simulink model "spec_avg_CRD"  (R2025b)
settings: Solver=FixedStepDiscrete  StartTime=0.0  StopTime=0.0005  FixedStep=1/Fs  RelTol=1e-3
undefined symbols (not defined in the file): Add, chirp_counts, chirp_outputs, FFT_LENGTH, Fs, h, N, Shift, specAvg, T, Ts
libraries: hdlsllib x5, dsphdlsigops2 x3, dsphdlmathfun2 x1, commutil2 x1, dsphdlxfrm2 x1
settings Model: MinMaxOverflowLogging=MinMaxAndOverflow  FPTRunName=BaselineRun  FPTShortcutValueString='{{},{''BaselineRun'',1,1,1,''BaselineRun'','''',{},''M'','''',''''},{''EmbeddedRun'',1,1,1,''EmbeddedRun'','''',{},''M'','''',''''},{''BaselineRun_2'',1,1,1,''BaselineRun_2'','''',{},''M'','''',''''},{''BaselineRun_3'',1,1,1,''BaselineRun_3'','''',{},''M'','''',''''},{''BaselineRun_4'',1,1,1,''BaselineRun_4'','''',{},''M'','''',''''},{''BaselineRun_5'',1,1,1,''BaselineRun_5'','''',{},''M'','''',''''}}'  Creator=caleb  LastModifiedBy=caleb
settings OptimizationCC: BlockReduction=off  DefaultParameterBehavior=Inlined  OptimizeBlockIOStorage=off  ReuseModelBlockBuffer=off  EnhancedBackFolding=on  PassReuseOutputArgsAs=Individual arguments  OptimizeBlockOrder=speed  DifferentSizesBufferReuse=on  EfficientTunableParamExpr=on
settings DebuggingCC: SignalRangeChecking=warning  SingleTaskRateTransMsg=error  ParameterTunabilityLossMsg=error
settings HardwareCC: TargetBitPerPointer=64.0  TargetBitPerSizeT=64.0  TargetBitPerPtrDiffT=64.0  TargetLongLongMode=on  TargetIntDivRoundTo=Zero  TargetEndianess=LittleEndian  TargetWordSize=64.0  TargetHWDeviceType=Generic->Custom  ProdEqTarget=off
settings SFSimCC: MATLABDynamicMemAlloc=off
settings RTWCC: SystemTargetFile=systemverilog_dpi_ert.tlc  TemplateMakefile=systemverilog_dpi_ert_default_tmf  GPUComputeCapability=3.5  Description=SystemVerilog DPI Component Generator
settings CodeAppCC: ForceParamTrailComments=on  IgnoreCustomStorageClasses=off  MaxIdLength=256.0  OperatorAnnotations=on  SimulinkDataObjDesc=on  SFDataObjDesc=on  InsertBlockDesc=on
settings DPIERTTargetCC: DPICustomizeSystemVerilogCode=off  DPISystemVerilogTemplate=svdpi_event.vgt  DPIReportRunTimeError=off  DPIScalarizePorts=off  DPIRunTimeErrorSeverity=Fatal  DPIGenerateTestBench=off  DPIFloatingPointTolerance=4.4409e-16  DPITestBenchSimulator=Siemens Questa/ModelSim  DPITestPointAccessFcnInterface=None  DPIFixedPointDataType=CompatibleCType  DPIPortConnection=Port list  DPICompositeDataType=Flattened  DPIComponentTemplateType=Sequential  DSAsUniqueAccess=off  ExtMode=off  ExtModeTransport=0.0  ExtModeStaticAlloc=off  ExtModeAutomaticAllocSize=on  ExtModeMaxTrigDuration=10.0  ExtModeStaticAllocSize=1000000.0  ExtModeTesting=off  ExtModeMexFile=ext_comm  ExtModeIntrfLevel=Level1  InlinedParameterPlacement=NonHierarchical  TargetOS=BareBoardExample  MultiInstanceErrorCode=Error  RootIOFormat=Part of model data structure  SubcomponentRootIOFormat=Auto  RTWCAPISignals=on  RTWCAPIParams=off  RTWCAPIStates=off  RTWCAPIRootIO=off  ERTSrcFileBannerTemplate=ert_code_template.cgt  ERTHdrFileBannerTemplate=ert_code_template.cgt  ERTDataSrcFileTemplate=ert_code_template.cgt  ERTDataHdrFileTemplate=ert_code_template.cgt  ERTCustomFileTemplate=example_file_process.tlc  EnableDataOwnership=off  SignalDisplayLevel=10.0  ParamTuneLevel=10.0  GlobalDataDefinition=Auto  DataDefinitionFile=global.c  GlobalDataReference=Auto  ERTFilePackagingFormat=Modular  RateTransitionBlockCode=Inline  DataReferenceFile=global.h  PreserveExpressionOrder=off  PreserveIfCondition=off  ConvertIfToSwitch=on  PreserveExternInFcnDecls=on  PreserveStaticInFcnDecls=on  SuppressUnreachableDefaultCases=on  EnableSignedLeftShifts=on  EnableSignedRightShifts=on  ImplementImageWithCVMat=off  IndentStyle=K&R  IndentSize=2  NewlineStyle=Default  MaxLineWidth=80.0  EnableUserReplacementTypes=off  MaxIdInt64=MAX_int64_T  MinIdInt64=MIN_int64_T  MaxIdUint64=MAX_uint64_T  MaxIdInt32=MAX_int32_T  MinIdInt32=MIN_int32_T  MaxIdUint32=MAX_uint32_T  MaxIdInt16=MAX_int16_T  MinIdInt16=MIN_int16_T  MaxIdUint16=MAX_uint16_T  MaxIdInt8=MAX_int8_T  MinIdInt8=MIN_int8_T  MaxIdUint8=MAX_uint8_T  BooleanTrueId=true  BooleanFalseId=false  MemSecPackage=--- None ---  MemSecDataConstants=Default  MemSecDataIO=Default  MemSecDataInternal=Default  MemSecDataParameters=Default  MemSecFuncInitTerm=Default  MemSecFuncExecute=Default  MemSecFuncSharedUtil=Default  GroupConstants=Default  GroupRootInputs=Default  GroupRootOutputs=Default  GroupInternal=Default  GroupParameters=Default  GroupDataTransfer=Default  GroupSharedLocalDataStores=Default  GroupInstanceSpecificParameters=Default  GroupModelData=Default  ArrayContainerType=C-style array  DynamicArrayContainerType=coder::array  TargetFcnLib=ansi_tfl_table_tmw.mat  GenFloatMathFcnCalls=NOT IN USE  TargetLangStandard=C89/C90 (ANSI)  CodeReplacementLibrary=None  UtilityFuncGeneration=Auto  MultiwordTypeDef=System defined  MultiwordLength=2048.0  DynamicStringBufferSize=256.0  GenerateFullHeader=on  InferredTypesCompatibility=off  GenerateSampleERTMain=off  GenerateTestInterfaces=off  ModelReferenceCompliant=on  ParMdlRefBuildCompliant=on  CompOptLevelCompliant=off  ConcurrentExecutionCompliant=off  IncludeMdlTerminateFcn=on  CombineOutputUpdateFcns=off  CombineSignalStateStructs=on  GroupInternalDataByFunction=off  SuppressErrorStatus=off  IncludeFileDelimiter=Auto  ERTCustomFileBanners=on  SupportAbsoluteTime=on  LogVarNameModifier=rt_  MatFileLogging=off  PreserveMATLABNamespacesInGeneratedCode=on  CodeInterfacePackaging=Reusable function  SubcomponentCodeInterfacePackaging=Reusable function  PurelyIntegerCode=off  SupportNonFinite=on  SupportComplex=on  SupportContinuousTime=on  SupportNonInlinedSFcns=on  RemoveDisableFunc=off  RemoveResetFunc=on  SupportVariableSizeSignals=off  ParenthesesLevel=Nominal  CastingMode=Nominal  MATLABClassNameForMDSCustomization=Simulink.SoftwareTarget.TargetSpecificTriggerConfigurationBase  ModelStepFunctionPrototypeControlCompliant=on  CPPClassGenCompliant=off  AutosarCompliant=off  MDXCompliant=off  GRTInterface=off  GenerateAllocFcn=on  UseToolchainInfoCompliant=on  GenerateSharedConstants=on  CoderGroups=[]  AccessMethods=[]  LookupTableObjectStructAxisOrder=1,2,3,4,...  LUTObjectStructOrderExplicitValues=Size,Breakpoints,Table  LUTObjectStructOrderEvenSpacing=Size,Breakpoints,Table  ArrayLayout=Column-major  UnsupportedSFcnMsg=error  ERTHeaderFileRootName=$R$E  ERTSourceFileRootName=$R$E  ERTDataFileRootName=$R_data  InstructionSetFMA=off  OptimizeReductions=off  LogToMDFFile=off

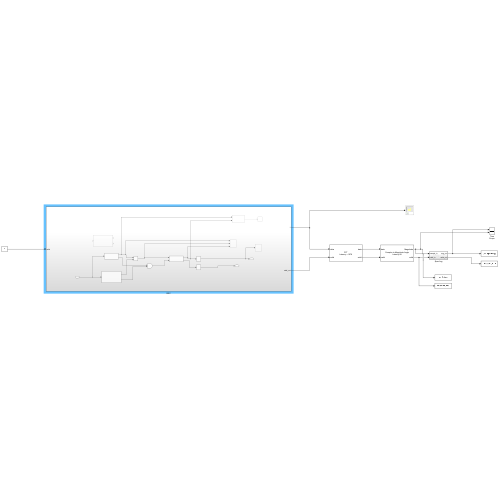
[thumbnail: Simulink's stored preview of the top-level diagram]
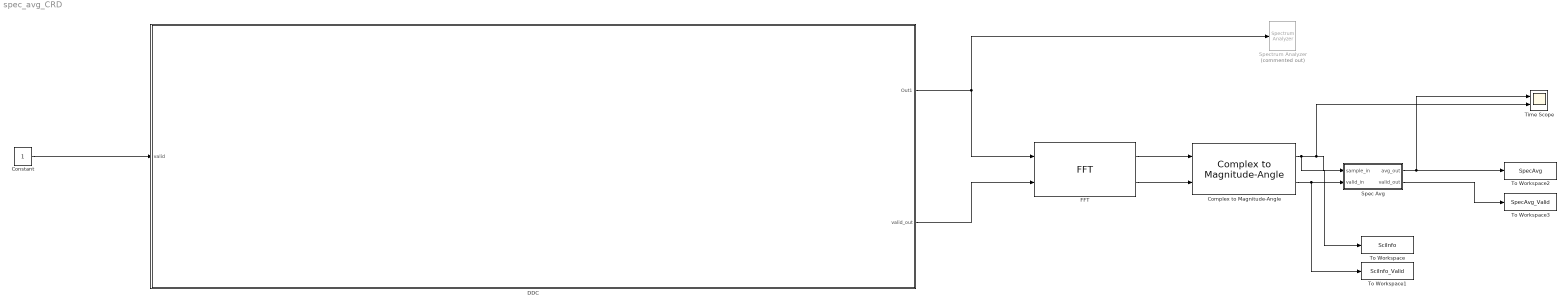
== system spec_avg_CRD ==
  Complex to Magnitude-Angle : dsphdlmathfun2/Complex to Magnitude-Angle  NumIterationsSource=Auto  NumIterations=10  OutputFormat=Magnitude  AngleFormat=Normalized  ScaleOutput=off  ScalingMethod=Shift-Add  SimulateUsing=Code generation
  Constant : Constant  OutDataTypeStr=boolean  SampleTime=Ts
  DDC : Subsystem
  FFT : dsphdlxfrm2/FFT  Architecture=Streaming Radix 2^2  FFTLengthSource=Property  FFTLength=FFT_LENGTH  FFTLengthMax=1024  ComplexMultiplication=Use 4 multipliers and 2 adders  BitReversedOutput=off  BitReversedInput=off  Normalize=off  SimulateUsing=Code generation  RoundingMethod=Floor  ResetInputPort=off  StartOutputPort=off  EndOutputPort=off
  Spec Avg : Subsystem
  Spectrum Analyzer : SpectrumAnalyzer  Commented=on  WindowPosition=[484.000000,227.000000,800.000000,500.000000,]  ScopeFrameLocation=window  WindowInvariantSamplesPerUpdate=on  YLimits=[-49.9819 21.9912]
  Time Scope : Scope  NumInputPorts=2
      settings: TimeUnits=Metric (based on Time Span)  ActiveDisplayYMinimum=-12388.774918989275  ActiveDisplayYMaximum=11609.175558970132  YLabel=Amplitude
  To Workspace : ToWorkspace  VariableName=SciInfo  SaveFormat=Timeseries  SampleTime=-1
  To Workspace1 : ToWorkspace  VariableName=SciInfo_Valid  SaveFormat=Timeseries  SampleTime=-1
  To Workspace2 : ToWorkspace  VariableName=SpecAvg  SaveFormat=Timeseries  SampleTime=-1
  To Workspace3 : ToWorkspace  VariableName=SpecAvg_Valid  SaveFormat=Timeseries  SampleTime=-1
  wires:
  Constant/1 -> DDC/1(valid)
  FFT/1 -> Complex to Magnitude-Angle/1
  DDC/1(Out1) -> FFT/1, Spectrum Analyzer/1
  DDC/2(valid_out) -> FFT/2
  FFT/2 -> Complex to Magnitude-Angle/2
  Complex to Magnitude-Angle/2 -> To Workspace1/1, Spec Avg/2(valid_in)
  Spec Avg/2(valid_out) -> To Workspace3/1
  Spec Avg/1(avg_out) -> Time Scope/1, To Workspace2/1
  Complex to Magnitude-Angle/1 -> Spec Avg/1(sample_in), Time Scope/2, To Workspace/1

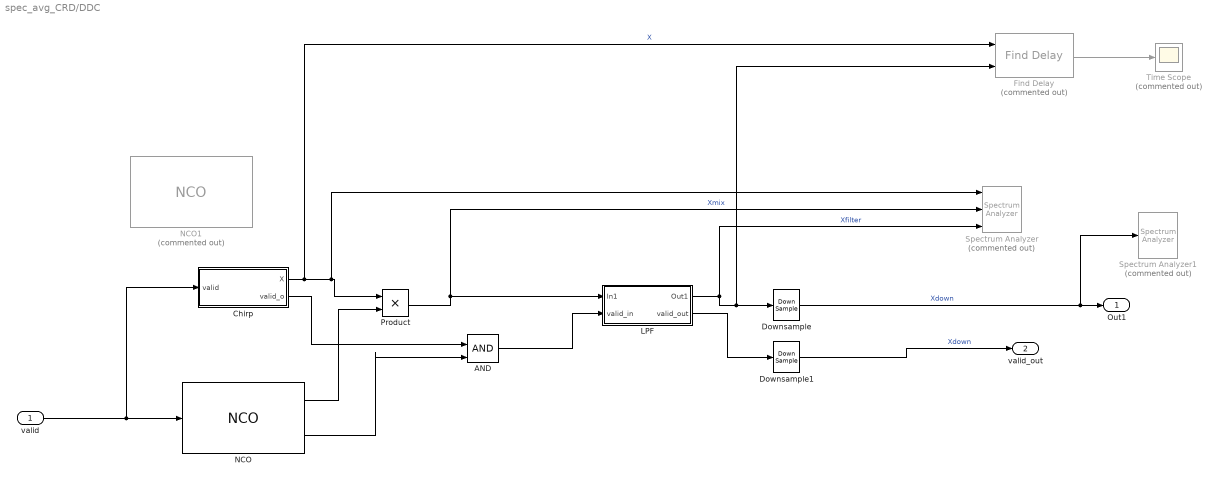
== system spec_avg_CRD/DDC ==
  valid : Inport
  AND : Logic  IconShape=distinctive  AllPortsSameDT=off  OutDataTypeStr=boolean
  Chirp : Subsystem
  Downsample : DownSample  RateOptions=Allow multirate processing
  Downsample1 : DownSample  RateOptions=Allow multirate processing
  Find Delay : commutil2/Find Delay  Commented=on  corrLength=100  chgSigOP=off  stopUpdate=off  numConstDelay=3
  LPF : Subsystem
  NCO : dsphdlsigops2/NCO  PhaseIncrementSource=Property  PhaseIncrement=phIncr  PhaseOffsetSource=Property  PhaseOffset=phOff  DitherSource=Property  NumDitherBits=ditherBits  SamplesPerFrame=1  LUTCompress=off  ResetAction=off  Waveform=Cosine  PhasePort=off  SimulateUsing=Code generation  AccumulatorWL=N  PhaseQuantization=on  NumQuantizerAccumulatorBits=Q  OutputDataType=Binary point scaling  OutputWL=16  OutputFL=14
  NCO1 : dsphdlsigops2/NCO  Commented=on  PhaseIncrementSource=Property  PhaseIncrement=phIncr  PhaseOffsetSource=Property  PhaseOffset=phOff  DitherSource=Property  NumDitherBits=ditherBits  SamplesPerFrame=1  LUTCompress=off  ResetAction=off  Waveform=Cosine  PhasePort=off  SimulateUsing=Code generation  AccumulatorWL=N  PhaseQuantization=on  NumQuantizerAccumulatorBits=Q  OutputDataType=Binary point scaling  OutputWL=16  OutputFL=14
  Product : Product  OutDataTypeStr=fixdt(1,16,14)
  Spectrum Analyzer : SpectrumAnalyzer  Commented=on  NumInputPorts=3  WindowPosition=[659 155 800 450]  Visible=on  SampleRate=60000000  Span=60000000  StartFrequency=-30000000  StopFrequency=30000000  AveragingMethod=Exponential  YLimits=[-111.52178032626103743,15.318431821757176436]  ShowLegend=on  AllowFFTLengthLessThanSamplesPerUpdate=on
  Spectrum Analyzer1 : SpectrumAnalyzer  Commented=on  WindowPosition=[33.8 11.8 800 450]  Visible=on  SampleRate=30000000  Span=30000000  StartFrequency=-15000000  StopFrequency=15000000  AveragingMethod=Exponential  YLimits=[-85.044423627277367927,9.5592900943282721471]  AllowFFTLengthLessThanSamplesPerUpdate=on
  Time Scope : Scope  Commented=on
      settings: TimeUnits=Metric (based on Time Span)  ActiveDisplayYMinimum=37.597540467169026  ActiveDisplayYMaximum=105.91635388327518  YLabel=Amplitude
  Out1 : Outport  VectorParamsAs1DForOutWhenUnconnected=off
  valid_out : Outport  Port=2  VectorParamsAs1DForOutWhenUnconnected=off
  wires:
  NCO/2 -> AND/2
  LPF/1(Out1) -> Find Delay/2, Downsample/1, Spectrum Analyzer/3  "Xfilter"
  Product/1 -> Spectrum Analyzer/2, LPF/1(In1)  "Xmix"
  valid/1 -> Chirp/1(valid), NCO/1
  NCO/1 -> Product/2
  Downsample/1 -> Out1/1, Spectrum Analyzer1/1  "Xdown"
  Chirp/1(X) -> Find Delay/1, Spectrum Analyzer/1, Product/1  "X"
  Find Delay/1 -> Time Scope/1
  LPF/2(valid_out) -> Downsample1/1
  Downsample1/1 -> valid_out/1  "Xdown"
  AND/1 -> LPF/2(valid_in)
  Chirp/2(valid_o) -> AND/1

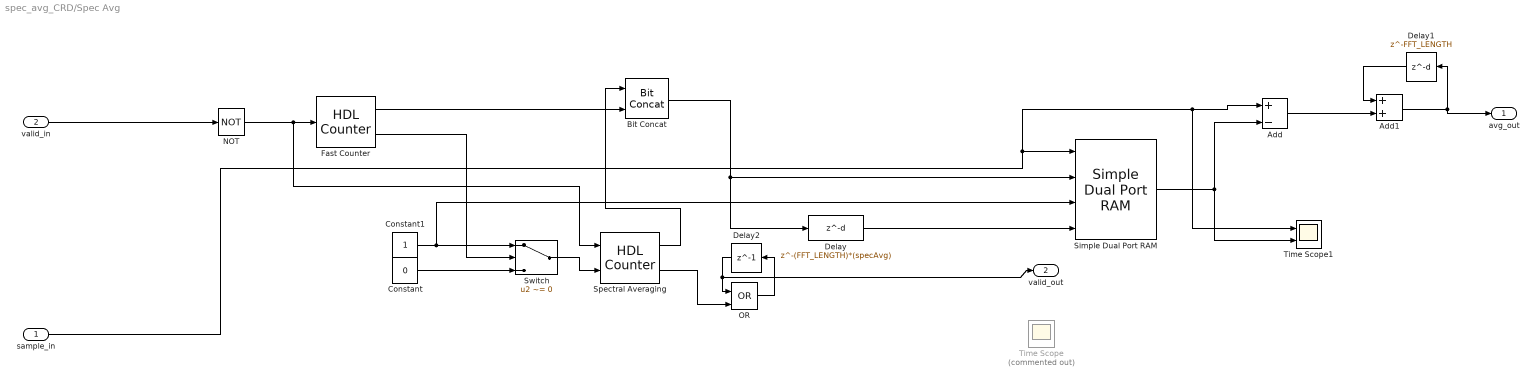
== system spec_avg_CRD/Spec Avg ==
  sample_in : Inport  OutDataTypeStr=fixdt(1,26,15)
  valid_in : Inport  Port=2
  Add : Sum  Inputs=+-  OutDataTypeStr=fixdt(1,16,7)
  Add1 : Sum  OutDataTypeStr=fixdt(1,32,4)  AccumDataTypeStr=fixdt(1,32,4)
  Bit Concat : hdlsllib/Logic and Bit Operations/Bit Concat  numInputs=2
  Constant : Constant  Value=0  OutDataTypeStr=boolean  SampleTime=2/Fs
  Constant1 : Constant  OutDataTypeStr=boolean  SampleTime=2/Fs
  Delay : Delay  DelayLength=(FFT_LENGTH)*(specAvg)
  Delay1 : Delay  DelayLength=FFT_LENGTH
  Delay2 : Delay  DelayLength=1
  Fast Counter : hdlsllib/Sources/HDL Counter  CountType=Modulo  CountInit=0  CountStep=1  CountMax=FFT_LENGTH-1  CountFromType=Initial value  CountFrom=0  CountResetPort=on  CountLoadPort=off  CountEnbPort=off  CountDirPort=off  CountHitOutputPort=on  CountDataType=Unsigned  CountWordLen=log2(FFT_LENGTH)  CountFracLen=0  CountSampTime=2/Fs
  NOT : Logic  Operator=NOT  IconShape=distinctive  AllPortsSameDT=off  OutDataTypeStr=boolean
  OR : Logic  Operator=OR  IconShape=distinctive  AllPortsSameDT=off  OutDataTypeStr=boolean
  Simple Dual Port RAM : hdlsllib/HDL RAMs/Simple Dual Port RAM  ram_size=ceil(log2(specAvg))+log2(FFT_LENGTH)
  Spectral Averaging : hdlsllib/Sources/HDL Counter  CountType=Modulo  CountInit=0  CountStep=1  CountMax=specAvg  CountFromType=Initial value  CountFrom=0  CountResetPort=on  CountLoadPort=off  CountEnbPort=on  CountDirPort=off  CountHitOutputPort=on  CountDataType=Unsigned  CountWordLen=ceil(log2(specAvg))  CountFracLen=0  CountSampTime=2/Fs
  Switch : Switch  Criteria=u2 ~= 0  SaturateOnIntegerOverflow=off  InputSameDT=off
  Time Scope : Scope  Commented=on
      settings: TimeUnits=Metric (based on Time Span)  ActiveDisplayYMinimum=-19.643385965811856  ActiveDisplayYMaximum=19.417275822629765  YLabel=Amplitude  DataLoggingVariableName=ScopeData2
  Time Scope1 : Scope  NumInputPorts=2
      settings: TimeUnits=Metric (based on Time Span)  ActiveDisplayYMinimum=-12.475021362304684  ActiveDisplayYMaximum=112.27519226074219  YLabel=Amplitude  DataLoggingVariableName=ScopeData3
  avg_out : Outport
  valid_out : Outport  Port=2  VectorParamsAs1DForOutWhenUnconnected=off
  wires:
  Switch/1 -> Spectral Averaging/2
  Fast Counter/2 -> Switch/2
  Constant/1 -> Switch/3
  Constant1/1 -> Simple Dual Port RAM/3, Switch/1
  Spectral Averaging/1 -> Bit Concat/1
  Fast Counter/1 -> Bit Concat/2
  Bit Concat/1 -> Simple Dual Port RAM/2, Delay/1
  sample_in/1 -> Simple Dual Port RAM/1, Add/1, Time Scope1/1
  Delay/1 -> Simple Dual Port RAM/4
  Simple Dual Port RAM/1 -> Time Scope1/2, Add/2
  Spectral Averaging/2 -> OR/2
  Delay2/1 -> OR/1, valid_out/1
  OR/1 -> Delay2/1
  Add/1 -> Add1/2
  Delay1/1 -> Add1/1
  Add1/1 -> avg_out/1, Delay1/1
  NOT/1 -> Spectral Averaging/1, Fast Counter/1
  valid_in/1 -> NOT/1

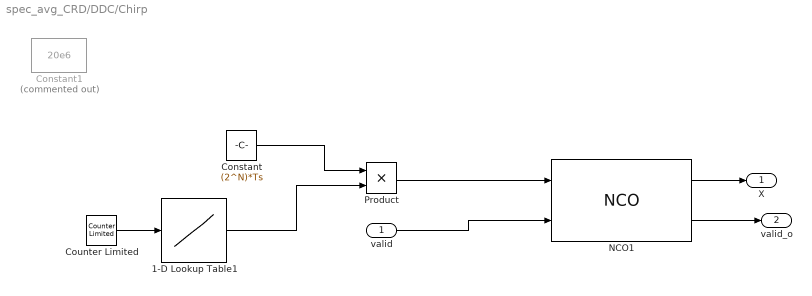
== system spec_avg_CRD/DDC/Chirp ==
  valid : Inport
  1-D Lookup Table1 : Lookup_n-D  NumberOfTableDimensions=1  LookupTableObject=''  BreakpointsForDimension1=chirp_counts  BreakpointsForDimension1FirstPoint=10  BreakpointsForDimension2FirstPoint=10  BreakpointsForDimension1Spacing=12  BreakpointsForDimension2Spacing=12  BreakpointsForDimension1DataTypeStr=uint16  IndexSearchMethod=Evenly spaced points  Table=chirp_outputs  TableDataTypeStr=uint32  InterpMethod=Flat  DiagnosticForOutOfRangeInput=Error  InternalRulePriority=Speed  OutDataTypeStr=uint32  RndMeth=Simplest  LockScale=on
  Constant : Constant  Value=(2^N)*Ts  OutDataTypeStr=fixdt(0,16,10)  SampleTime=1/Fs
  Constant1 : Constant  Commented=on  Value=20e6
  Counter Limited : hdlsllib/Sources/Counter Limited  uplimit=T/Ts  tsamp=1/Fs
  NCO1 : dsphdlsigops2/NCO  PhaseIncrementSource=Input port  PhaseIncrement=phIncr  PhaseOffsetSource=Property  PhaseOffset=phOff  DitherSource=Property  NumDitherBits=ditherBits  SamplesPerFrame=1  LUTCompress=off  ResetAction=off  Waveform=Cosine  PhasePort=off  SimulateUsing=Code generation  AccumulatorWL=N  PhaseQuantization=on  NumQuantizerAccumulatorBits=Q  OutputDataType=Binary point scaling  OutputWL=16  OutputFL=14
  Product : Product  OutDataTypeStr=uint32  LockScale=on
  X : Outport
  valid_o : Outport  Port=2
  wires:
  Constant/1 -> Product/1
  valid/1 -> NCO1/2
  NCO1/2 -> valid_o/1
  NCO1/1 -> X/1
  Product/1 -> NCO1/1
  Counter Limited/1 -> 1-D Lookup Table1/1
  1-D Lookup Table1/1 -> Product/2

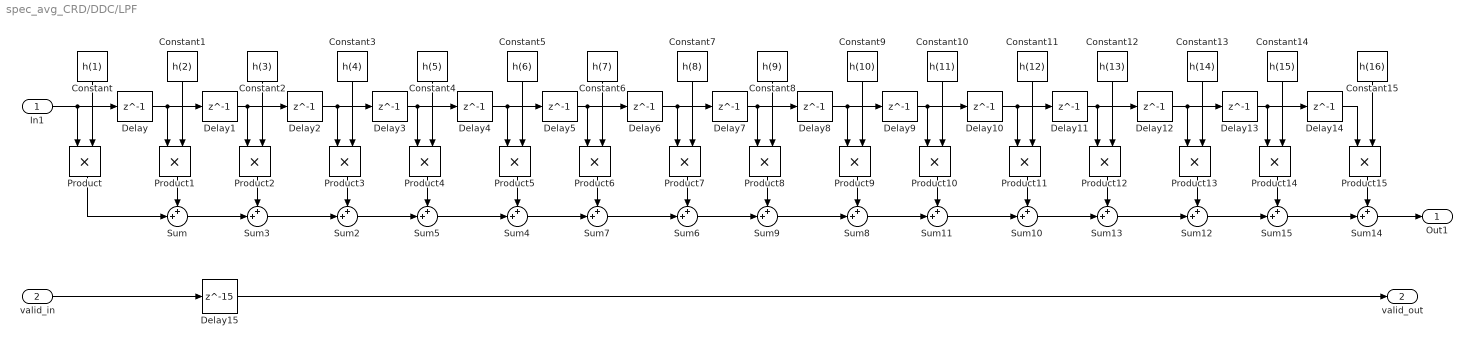
== system spec_avg_CRD/DDC/LPF ==
  In1 : Inport  OutDataTypeStr=fixdt(1,16,14)
  valid_in : Inport  Port=2  OutDataTypeStr=boolean
  Constant : Constant  Value=h(1)  OutDataTypeStr=fixdt(1,16,4)  SampleTime=1/Fs
  Constant1 : Constant  Value=h(2)  OutDataTypeStr=fixdt(1,16,25)  SampleTime=1/Fs
  Constant10 : Constant  Value=h(11)  OutDataTypeStr=fixdt(0,16,19)  SampleTime=1/Fs
  Constant11 : Constant  Value=h(12)  OutDataTypeStr=fixdt(0,16,23)  SampleTime=1/Fs
  Constant12 : Constant  Value=h(13)  OutDataTypeStr=fixdt(1,16,21)  SampleTime=1/Fs
  Constant13 : Constant  Value=h(14)  OutDataTypeStr=fixdt(1,16,22)  SampleTime=1/Fs
  Constant14 : Constant  Value=h(15)  OutDataTypeStr=fixdt(1,16,25)  SampleTime=1/Fs
  Constant15 : Constant  Value=h(16)  OutDataTypeStr=fixdt(1,16,4)  SampleTime=1/Fs
  Constant2 : Constant  Value=h(3)  OutDataTypeStr=fixdt(1,16,22)  SampleTime=1/Fs
  Constant3 : Constant  Value=h(4)  OutDataTypeStr=fixdt(1,16,21)  SampleTime=1/Fs
  Constant4 : Constant  Value=h(5)  OutDataTypeStr=fixdt(0,16,23)  SampleTime=1/Fs
  Constant5 : Constant  Value=h(6)  OutDataTypeStr=fixdt(0,16,19)  SampleTime=1/Fs
  Constant6 : Constant  Value=h(7)  OutDataTypeStr=fixdt(0,16,18)  SampleTime=1/Fs
  Constant7 : Constant  Value=h(8)  OutDataTypeStr=fixdt(0,16,17)  SampleTime=1/Fs
  Constant8 : Constant  Value=h(9)  OutDataTypeStr=fixdt(0,16,17)  SampleTime=1/Fs
  Constant9 : Constant  Value=h(10)  OutDataTypeStr=fixdt(0,16,18)  SampleTime=1/Fs
  Delay{,1..14} (15 alike) : Delay  DelayLength=1  InitialCondition=0  UseCircularBuffer=on
  Delay15 : Delay  DelayLength=15
  Product : Product  OutDataTypeStr=fixdt(1,16,4)
  Product1 : Product  OutDataTypeStr=fixdt(1,16,25)
  Product10 : Product  OutDataTypeStr=fixdt(1,16,18)
  Product{2,4,11,13} (4 alike) : Product  OutDataTypeStr=fixdt(1,16,22)
  Product12 : Product  OutDataTypeStr=fixdt(1,16,21)
  Product14 : Product  OutDataTypeStr=fixdt(1,16,25)
  Product15 : Product  OutDataTypeStr=fixdt(1,16,4)
  Product3 : Product  OutDataTypeStr=fixdt(1,16,21)
  Product5 : Product  OutDataTypeStr=fixdt(1,16,18)
  Product6 : Product  OutDataTypeStr=fixdt(1,16,17)
  Product7 : Product  OutDataTypeStr=fixdt(1,16,16)
  Product8 : Product  OutDataTypeStr=fixdt(1,16,16)
  Product9 : Product  OutDataTypeStr=fixdt(1,16,17)
  Sum : Sum  Inputs=++|  OutDataTypeStr=fixdt(1,16,25)
  Sum{8,10..15} (7 alike) : Sum  Inputs=++|  OutDataTypeStr=fixdt(1,16,15)
  Sum2 : Sum  Inputs=++|  OutDataTypeStr=fixdt(1,16,21)
  Sum3 : Sum  Inputs=++|  OutDataTypeStr=fixdt(1,16,22)
  Sum4 : Sum  Inputs=++|  OutDataTypeStr=fixdt(1,16,18)
  Sum5 : Sum  Inputs=++|  OutDataTypeStr=fixdt(1,16,21)
  Sum6 : Sum  Inputs=++|  OutDataTypeStr=fixdt(1,16,16)
  Sum7 : Sum  Inputs=++|  OutDataTypeStr=fixdt(1,16,17)
  Sum9 : Sum  Inputs=++|  OutDataTypeStr=fixdt(1,16,16)
  Out1 : Outport
  valid_out : Outport  Port=2  VectorParamsAs1DForOutWhenUnconnected=off
  wires:
  In1/1 -> Delay/1, Product/1
  Delay/1 -> Product1/1, Delay1/1
  Constant/1 -> Product/2
  Constant1/1 -> Product1/2
  Product1/1 -> Sum/1
  Product/1 -> Sum/2
  Constant2/1 -> Product2/2
  Delay1/1 -> Delay2/1, Product2/1
  Product2/1 -> Sum3/1
  Delay2/1 -> Product3/1, Delay3/1
  Sum3/1 -> Sum2/2
  Constant3/1 -> Product3/2
  Product3/1 -> Sum2/1
  Constant4/1 -> Product4/2
  Delay3/1 -> Delay4/1, Product4/1
  Product4/1 -> Sum5/1
  Delay4/1 -> Product5/1, Delay5/1
  Sum5/1 -> Sum4/2
  Constant5/1 -> Product5/2
  Product5/1 -> Sum4/1
  Constant6/1 -> Product6/2
  Delay5/1 -> Delay6/1, Product6/1
  Product6/1 -> Sum7/1
  Delay6/1 -> Product7/1, Delay7/1
  Sum7/1 -> Sum6/2
  Constant7/1 -> Product7/2
  Product7/1 -> Sum6/1
  Constant8/1 -> Product8/2
  Delay7/1 -> Delay8/1, Product8/1
  Product8/1 -> Sum9/1
  Delay8/1 -> Product9/1, Delay9/1
  Sum9/1 -> Sum8/2
  Constant9/1 -> Product9/2
  Product9/1 -> Sum8/1
  Constant10/1 -> Product10/2
  Delay9/1 -> Delay10/1, Product10/1
  Product10/1 -> Sum11/1
  Delay10/1 -> Product11/1, Delay11/1
  Sum11/1 -> Sum10/2
  Constant11/1 -> Product11/2
  Product11/1 -> Sum10/1
  Constant12/1 -> Product12/2
  Delay11/1 -> Delay12/1, Product12/1
  Product12/1 -> Sum13/1
  Delay12/1 -> Product13/1, Delay13/1
  Sum13/1 -> Sum12/2
  Constant13/1 -> Product13/2
  Product13/1 -> Sum12/1
  Constant14/1 -> Product14/2
  Delay13/1 -> Delay14/1, Product14/1
  Product14/1 -> Sum15/1
  Delay14/1 -> Product15/1
  Sum15/1 -> Sum14/2
  Constant15/1 -> Product15/2
  Product15/1 -> Sum14/1
  Sum12/1 -> Sum15/2
  Sum10/1 -> Sum13/2
  Sum8/1 -> Sum11/2
  Sum6/1 -> Sum9/2
  Sum4/1 -> Sum7/2
  Sum2/1 -> Sum5/2
  Sum/1 -> Sum3/2
  Sum14/1 -> Out1/1
  valid_in/1 -> Delay15/1
  Delay15/1 -> valid_out/1
